simulink subsystem "SteeringSystem"  (R2023b)
settings: Solver=VariableStepAuto  StartTime=0.0  StopTime=10.0  RelTol=1e-3
settings Model: Creator=konur  LastModifiedBy=konur

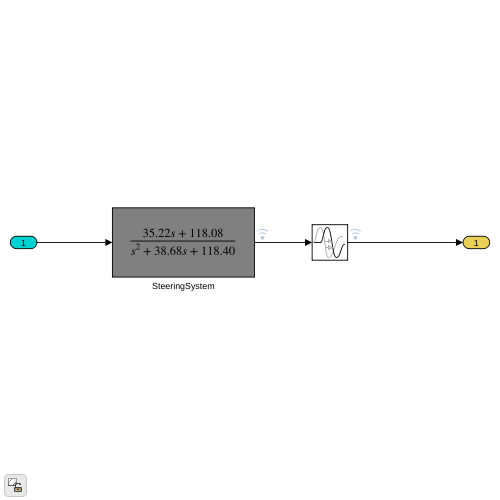
[thumbnail: Simulink's stored preview of the top-level diagram]
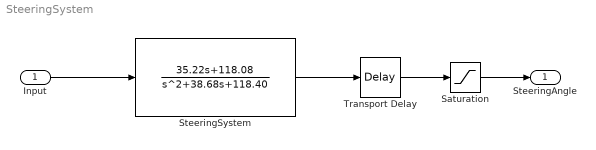
== system SteeringSystem ==
  Input : Inport
  Saturation : Saturate  UpperLimit=pi/5  LowerLimit=-pi/5
  SteeringSystem : TransferFcn  Numerator=[35.22,118.08]  Denominator=[1,38.68,118.40]  ContinuousStateAttributes="\"SteeringAngle\""
  Transport Delay : TransportDelay  DelayTime=0.05
  SteeringAngle : Outport
  wires:
  Transport Delay/1 -> Saturation/1
  SteeringSystem/1 -> Transport Delay/1
  Input/1 -> SteeringSystem/1
  Saturation/1 -> SteeringAngle/1
